simulink model "temperatura budynku"  (R2025b)
settings: Solver=ode23  StartTime=0.0  StopTime=20000  RelTol=1e-3
InitFcn:
  | a = 3; b = 3; h = 3.5;
  | c = 1000.5;
  | ro=1.3413;
  | m = a*b*h*ro;
  | A=2*a*h+2*b*h+a*b;
  | k=2;P=4500;
libraries: slpidlib x1
settings Model: Creator=Student  LastModifiedBy=maciuś

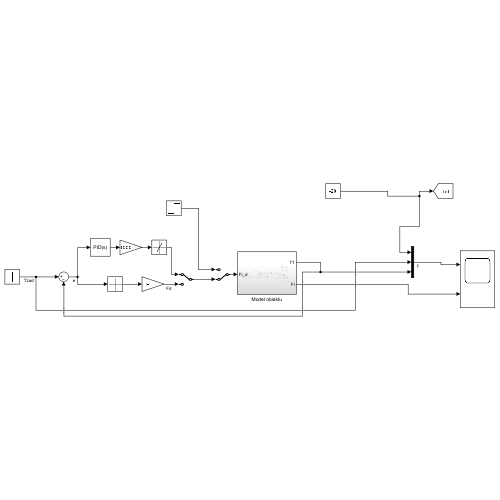
[thumbnail: Simulink's stored preview of the top-level diagram]
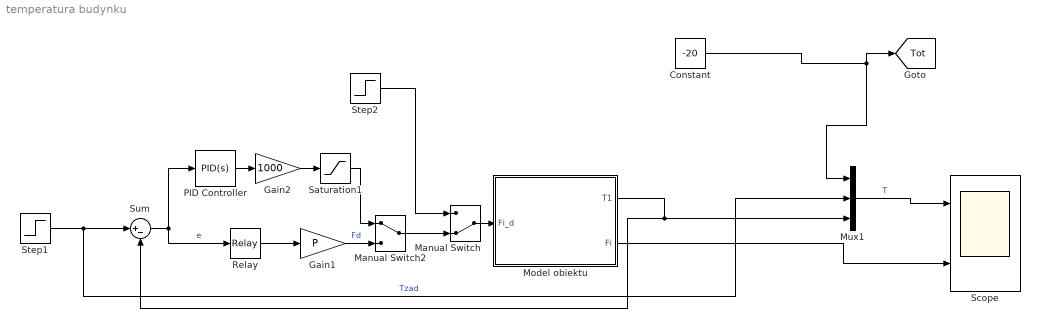
== system temperatura budynku ==
  Constant : Constant  Value=-20
  Gain1 : Gain  Gain=P
  Gain2 : Gain  Gain=1000
  Manual Switch : ManualSwitch  CurrentSetting=0
  Manual Switch2 : ManualSwitch
  Model obiektu : Subsystem
  Mux1 : Mux  Inputs=3
  PID Controller : slpidlib/PID Controller  Controller=PID  Form=Parallel  TimeDomain=Continuous-time  UseExternalTs=off  SampleTime=-1  IntegratorMethod=Forward Euler  FilterMethod=Forward Euler  ControllerParametersSource=internal  P=24  I=94  UseKiTs=off  D=23.5  UseExternalDerivativeSource=off  N=100  UseFilter=on  TunerSelectOption=Transfer Function Based (PID Tuner App)  InitialConditionSource=internal  InitialConditionForIntegrator=0  InitialConditionForFilter=0  DifferentiatorICPrevScaledInput=0  ExternalReset=none  TrackingMode=off  Kt=1  LimitOutput=off  SatLimitsSource=internal  UpperSaturationLimit=inf  LowerSaturationLimit=-inf  LinearizeAsGain=on  AntiWindupMode=none  Kb=1  LimitIntegrator=off  UpperIntegratorSaturationLimit=inf  LowerIntegratorSaturationLimit=-inf  POutMin=[]  POutMax=[]  IOutMin=[]  IOutMax=[]  DOutMin=[]  DOutMax=[]  NOutMin=[]  NOutMax=[]  SumOutMin=[]  SumOutMax=[]  SaturationOutMin=[]  SaturationOutMax=[]  PParamMin=[]  PParamMax=[]  IParamMin=[]  IParamMax=[]  DParamMin=[]  DParamMax=[]  NParamMin=[]  NParamMax=[]  KbParamMin=[]  KbParamMax=[]  KtParamMin=[]  KtParamMax=[]  KbOutMin=[]  KbOutMax=[]  KtOutMin=[]  KtOutMax=[]  IntegratorOutMin=[]  IntegratorOutMax=[]  FilterOutMin=[]  FilterOutMax=[]  SumI1OutMin=[]  SumI1OutMax=[]  SumI2OutMin=[]  SumI2OutMax=[]  SumI3OutMin=[]  SumI3OutMax=[]  SumI4OutMin=[]  SumI4OutMax=[]  SumDOutMin=[]  SumDOutMax=[]  DifferentiatorOutMin=[]  DifferentiatorOutMax=[]  FilterDiffOutCoefMin=[]  FilterDiffOutCoefMax=[]  ReciprocalOutMin=[]  ReciprocalOutMax=[]  SumDenOutMin=[]  SumDenOutMax=[]  SumNumOutMin=[]  SumNumOutMax=[]  DivideOutMin=[]  DivideOutMax=[]  UdiffTsProdOutMin=[]  UdiffTsProdOutMax=[]  NTsProdOutMin=[]  NTsProdOutMax=[]  UintegralTsProdOutMin=[]  UintegralTsProdOutMax=[]  UngainTsProdOutMin=[]  UngainTsProdOutMax=[]  ClampingZeroOutDataTypeStr=Inherit: Inherit via back propagation  ClampingZeroOutMin=[]  ClampingZeroOutMax=[]  FilterDenConstantOutDataTypeStr=Inherit: Inherit via back propagation  FilterDenConstantOutMin=[]  FilterDenConstantOutMax=[]  PCopyOutDataTypeStr=Inherit: Inherit via back propagation  PCopyOutMin=[]  PCopyOutMax=[]  NCopyOutDataTypeStr=Inherit: Inherit via back propagation  NCopyOutMin=[]  NCopyOutMax=[]  IntegratorContinuousStateAttributes=''  IntegratorStateMustResolveToSignalObject=off  IntegratorRTWStateStorageClass=Auto  FilterContinuousStateAttributes=''  FilterStateMustResolveToSignalObject=off  FilterRTWStateStorageClass=Auto  ParallelPVariant=InternalParameters  IdealPVariant=Disabled  IVariant=InternalParameters  DVariant=InternalParameters  IntegratorVariant=Continuous  SatVariant=Disabled  AWVariant=Passthrough  PCopyVariant=Disabled  TRVariant=Disabled  FdbkBlocksVariant=Forward  IdealPFdbkVariant=Disabled  SatFdbkVariant=Disabled  DerivativeFilterVariant=ContFilter  NVariant=InternalParameters  NCopyVariant=Disabled  FilterICVariant=InternalICsFilter  IntegratorICVariant=InternalICs  ExternalResetVariant=Disabled  TRSumVariant=Passthrough  SumFdbkVariant=Disabled  SumVariant=Sum_PID  TsampFilterVariant=InternalTs  TsampNgainVariant=Passthrough  TsampIntegralVariant=Disabled_SignalSpec  ExternalSaturationOutDataTypeStr=Inherit: Same as second input  DerivativeSourceVariant=ErrorSignal  PreIntVariant=InternalPreInt
  Relay : Relay  OnSwitchValue=2  OffSwitchValue=-2
  Saturation1 : Saturate  UpperLimit=P  LowerLimit=0
  Scope : Scope  NumInputPorts=2
      settings: ActiveDisplayYMinimum=-25.514705240976948  ActiveDisplayYMaximum=29.632352869879927
  Step1 : Step  Time=3600*2  Before=-20  After=19  SampleTime=0
  Step2 : Step  Time=3600*2  After=P  SampleTime=0
  Sum : Sum  Inputs=|+-
  tag scope: Tot=global
  wires:
  Sum/1 -> PID Controller/1, Relay/1  "e"
  Relay/1 -> Gain1/1
  Step2/1 -> Manual Switch/1
  Manual Switch/1 -> Model obiektu/1(Fi_d)
  Model obiektu/1(T1) -> Sum/2, Mux1/3
  Model obiektu/2(Fi) -> Scope/2
  Mux1/1 -> Scope/1  "T"
  Step1/1 -> Mux1/2, Sum/1  "Tzad"
  Constant/1 -> [Tot], Mux1/1
  Manual Switch2/1 -> Manual Switch/2
  Gain1/1 -> Manual Switch2/2  "Fd"
  PID Controller/1 -> Gain2/1
  Gain2/1 -> Saturation1/1
  Saturation1/1 -> Manual Switch2/1

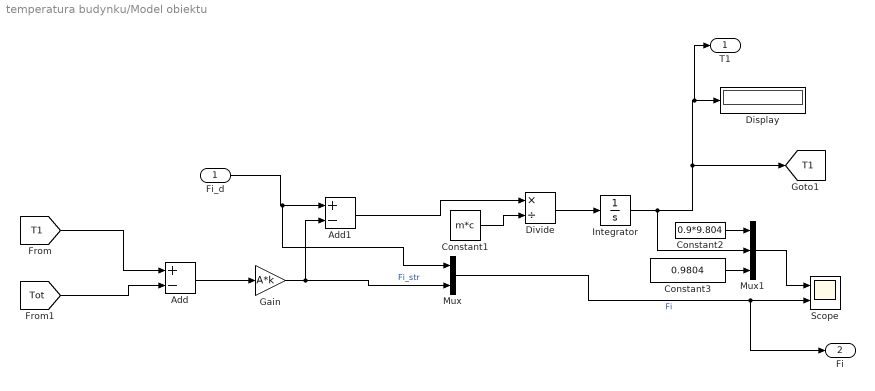
== system temperatura budynku/Model obiektu ==
  Fi_d : Inport
  Add : Sum  Inputs=+-
  Add1 : Sum  Inputs=+-
  Constant1 : Constant  Value=m*c
  Constant2 : Constant  Value=0.9*9.804
  Constant3 : Constant  Value=0.9804
  Display : Display
  Divide : Product  Inputs=*/
  Gain : Gain  Gain=A*k
  Integrator : Integrator
  Mux : Mux  Inputs=2
  Mux1 : Mux  Inputs=3
  Scope : Scope  NumInputPorts=2
      settings: ActiveDisplayYMinimum=-25.124999358627885  ActiveDisplayYMaximum=26.124999928738369
  T1 : Outport
  Fi : Outport  Port=2
  tag scope: T1=global
  wires:
  Mux/1 -> Fi/1, Scope/2  "Fi"
  [T1] -> Add/1
  Gain/1 -> Add1/2, Mux/2  "Fi_str"
  Divide/1 -> Integrator/1
  Add1/1 -> Divide/1
  Fi_d/1 -> Mux/1, Add1/1
  Integrator/1 -> Mux1/2, T1/1, Display/1, [T1]
  Add/1 -> Gain/1
  Constant1/1 -> Divide/2
  Mux1/1 -> Scope/1
  Constant3/1 -> Mux1/3
  Constant2/1 -> Mux1/1
  [Tot] -> Add/2
